simulink model "Formula_fuerza_gravedad"  (R2023a)
settings: Solver=FixedStepAuto  StartTime=0.0  StopTime=20E6  FixedStep=100  RelTol=1e-3
undefined symbols (not defined in the file or in its folder): G, M, R
libraries: simulink x1
settings Model: Creator=Nacho Andrade  LastModifiedBy=Nacho Andrade

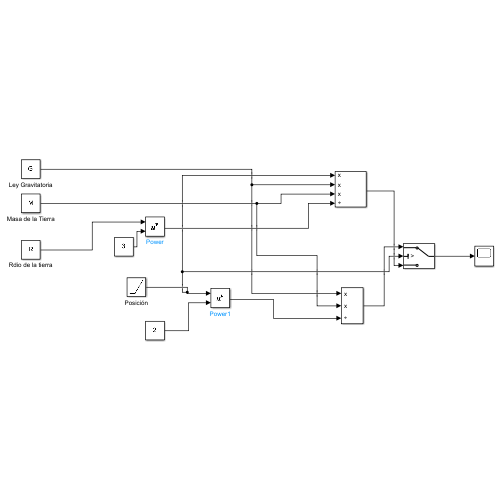
[thumbnail: Simulink's stored preview of the top-level diagram]
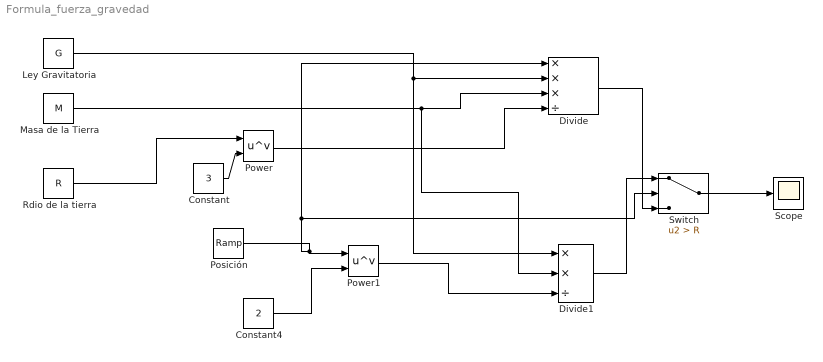
== system Formula_fuerza_gravedad ==
  Constant : Constant  Value=3
  Constant4 : Constant  Value=2
  Divide : Product  Inputs=***/
  Divide1 : Product  Inputs=**/
  Ley Gravitatoria : Constant  Value=G
  Masa de la Tierra : Constant  Value=M
  Posición : simulink/Sources/Ramp  slope=1  start=0  InitialOutput=0
  Power : Math  Operator=pow
  Power1 : Math  Operator=pow
  Rdio de la tierra : Constant  Value=R
  Scope : Scope
  Switch : Switch  Criteria=u2 > Threshold  Threshold=R  SaturateOnIntegerOverflow=off  InputSameDT=off
  wires:
  Constant/1 -> Power/2
  Rdio de la tierra/1 -> Power/1
  Power/1 -> Divide/4
  Constant4/1 -> Power1/2
  Posición/1 -> Power1/1, Switch/2, Divide/1
  Ley Gravitatoria/1 -> Divide1/1, Divide/2
  Masa de la Tierra/1 -> Divide1/2, Divide/3
  Power1/1 -> Divide1/3
  Divide1/1 -> Switch/1
  Divide/1 -> Switch/3
  Switch/1 -> Scope/1
